simulink model "sim"  (R2020a)
settings: Solver=VariableStepAuto  StartTime=0.0  StopTime=10.0  RelTol=1e-3
undefined symbols (not defined in the file): A, An, B, Bn, C, K_lqr, Ln, P_0, Q_n, R_n, Ts, x_0, x_kalman
libraries: simulink_extras x2
settings Model: Creator=Artis  LastModifiedBy=Artis

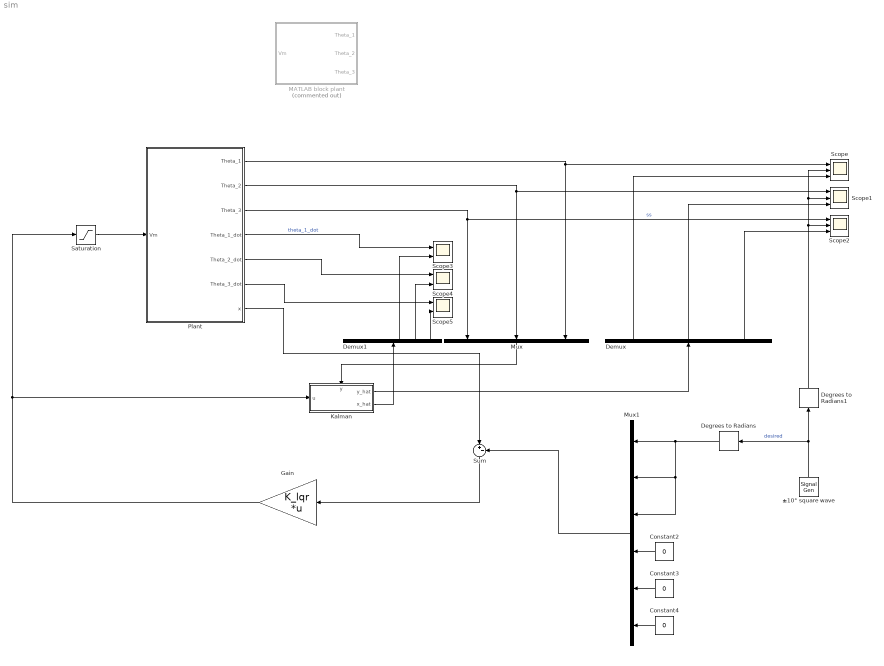
== system sim ==
  Constant2 : Constant  Value=0
  Constant3 : Constant  Value=0
  Constant4 : Constant  Value=0
  Degrees to Radians : simulink_extras/Transformations/Degrees to Radians
  Degrees to Radians1 : simulink_extras/Transformations/Degrees to Radians
  Demux : Demux  Outputs=3
  Demux1 : Demux  Outputs=6
  Gain : Gain  Gain=K_lqr  Multiplication=Matrix(K*u) (u vector)
  Kalman : Subsystem
      settings: PortSchema="{\"entries\":[{\"content\":{\"sides\":[{\"content\":{\"connectorIds\":[\"In1\"]},\"type\":\"ConnectorPlacement.EquallySpacedRectSide\",\"uuid\":\"62bff884-1764-4624-86bb-c0f466d25cc0\"},{\"content\":{\"connectorIds\":[\"Out1\",\"Out2\"],\"side\":\"RIGHT\"},\"type\":\"ConnectorPlacement.EquallySpacedRectSide\",\"uuid\":\"eceabb9a-6e11-42f6-82ff-ae26c39c3440\"},{\"content\":{\"connectorIds\":[\"In2\"],\"side\":\"TOP\"},\"type\":\"ConnectorPlacement.EquallySpacedRectSide\",\"uuid\":\"6bdeda42-7cc5-45d4-ac99-29c27164ef4c\"}]},\"type\":\"ConnectorPlacement.EquallySpacedConnector\",\"uuid\":\"cdaf1b78-b767-40c4-a6aa-db1d943e4267\"}],\"packageUris\":[\"http://schema.mathworks.com/mf0/Connector/19700101\"],\"version\":\"1.0\"}"
  MATLAB block plant : Subsystem  Commented=on
  Mux : Mux  Inputs=3
  Mux1 : Mux  Inputs=6
  Plant : Subsystem
  Saturation : Saturate  UpperLimit=6  LowerLimit=-6
  Scope : Scope  NumInputPorts=3
  Scope1 : Scope  NumInputPorts=3
  Scope2 : Scope  NumInputPorts=3
  Scope3 : Scope  NumInputPorts=2
  Scope4 : Scope  NumInputPorts=2
  Scope5 : Scope  NumInputPorts=2
  Sum : Sum  Inputs=|+-
  ±10° square wave : SignalGenerator  WaveForm=square  Amplitude=10  Units=rad/sec
  wires:
  Plant/1(Theta_1) -> Scope/1, Mux/3
  Plant/2(Theta_2) -> Mux/2, Scope1/1
  Plant/3(Theta_3) -> Mux/1, Scope2/1  "ss"
  Gain/1 -> Kalman/1(u), Saturation/1
  ±10° square wave/1 -> Degrees to Radians1/1, Degrees to Radians/1  "desired"
  Mux/1 -> Kalman/2(y)
  Kalman/1(y_hat) -> Demux/1
  Demux/1 -> Scope/3
  Demux/2 -> Scope1/3
  Demux/3 -> Scope2/3
  Plant/4(Theta_1_dot) -> Scope3/1  "theta_1_dot"
  Plant/5(Theta_2_dot) -> Scope4/1
  Plant/6(Theta_3_dot) -> Scope5/1
  Demux1/4 -> Scope3/2
  Demux1/5 -> Scope4/2
  Demux1/6 -> Scope5/2
  Kalman/2(x_hat) -> Demux1/1
  Sum/1 -> Gain/1
  Mux1/1 -> Sum/2
  Constant2/1 -> Mux1/4
  Constant3/1 -> Mux1/5
  Constant4/1 -> Mux1/6
  Plant/7(x) -> Sum/1
  Degrees to Radians/1 -> Mux1/3, Mux1/2, Mux1/1
  Saturation/1 -> Plant/1(Vm)
  Degrees to Radians1/1 -> Scope/2, Scope1/2, Scope2/2

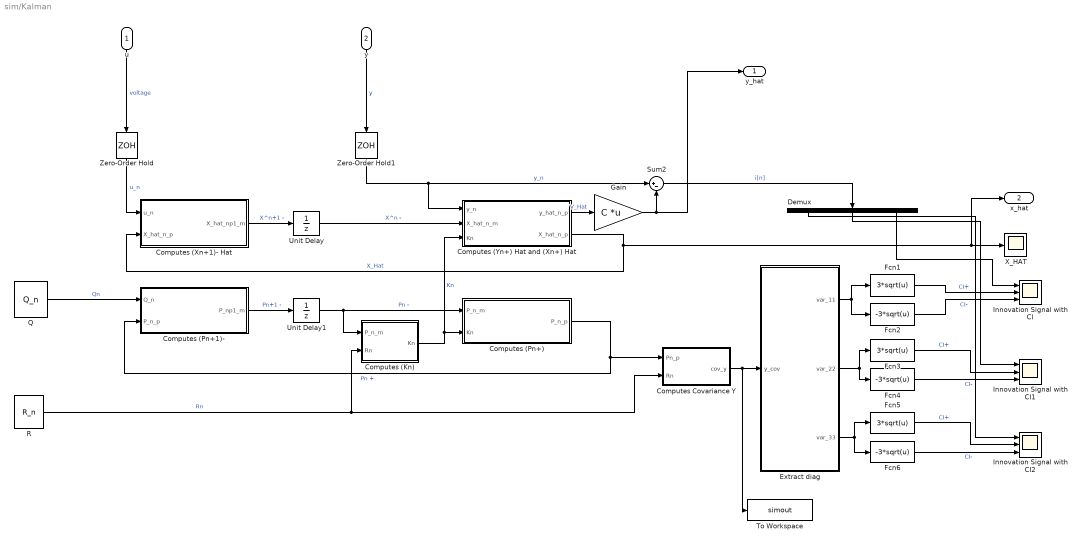
== system sim/Kalman ==
  u : Inport
  y : Inport  Port=2
  Computes (Kn) : MATLAB Function  TreatAsAtomicUnit=on
  Computes (Pn+) : MATLAB Function  TreatAsAtomicUnit=on
  "Computes (Pn+1)- " : MATLAB Function  TreatAsAtomicUnit=on
  Computes (Xn+1)- Hat : MATLAB Function  TreatAsAtomicUnit=on
  Computes (Yn+) Hat and (Xn+) Hat : MATLAB Function  TreatAsAtomicUnit=on
  Computes Covariance Y : MATLAB Function  TreatAsAtomicUnit=on
  Demux : Demux  Outputs=3
  Extract diag : MATLAB Function  TreatAsAtomicUnit=on
  Fcn1 : Fcn  Expr=3*sqrt(u)
  Fcn2 : Fcn  Expr=-3*sqrt(u)
  Fcn3 : Fcn  Expr=3*sqrt(u)
  Fcn4 : Fcn  Expr=-3*sqrt(u)
  Fcn5 : Fcn  Expr=3*sqrt(u)
  Fcn6 : Fcn  Expr=-3*sqrt(u)
  Gain : Gain  Gain=C  Multiplication=Matrix(K*u) (u vector)
  Innovation Signal with CI : Scope  NumInputPorts=3
  Innovation Signal with CI1 : Scope  NumInputPorts=3
  Innovation Signal with CI2 : Scope  NumInputPorts=3
  Q : Constant  Value=Q_n
  R : Constant  Value=R_n
  Sum2 : Sum  Inputs=|+-
  To Workspace : ToWorkspace  VariableName=simout  SampleTime=-1
  Unit Delay : UnitDelay  InitialCondition=x_kalman  SampleTime=Ts  HasFrameUpgradeWarning=on
  Unit Delay1 : UnitDelay  InitialCondition=P_0  SampleTime=Ts  HasFrameUpgradeWarning=on
  X_HAT : Scope
  Zero-Order Hold : ZeroOrderHold  SampleTime=Ts
  Zero-Order Hold1 : ZeroOrderHold  SampleTime=Ts
  y_hat : Outport
  x_hat : Outport  Port=2
  wires:
  Zero-Order Hold/1 -> Computes (Xn+1)- Hat/1(u_n)  "u_n"
  Fcn2/1 -> Innovation Signal with CI/3  "CI-"
  Unit Delay1/1 -> Computes (Pn+)/1(P_n_m), Computes (Kn)/1(P_n_m)  "Pn -"
  Computes (Xn+1)- Hat/1(X_hat_np1_m) -> Unit Delay/1  "X^n+1 -"
  R/1 -> Computes (Kn)/2(Rn), Computes Covariance Y/2(Rn)  "Rn"
  Computes (Kn)/1(Kn) -> Computes (Yn+) Hat and (Xn+) Hat/3(Kn), Computes (Pn+)/2(Kn)  "Kn"
  Fcn1/1 -> Innovation Signal with CI/2  "CI+"
  Sum2/1 -> Demux/1  "i[n]"
  u/1 -> Zero-Order Hold/1  "voltage"
  Computes (Yn+) Hat and (Xn+) Hat/1(y_hat_n_p) -> Gain/1  "V_Hat"
  Unit Delay/1 -> Computes (Yn+) Hat and (Xn+) Hat/2(X_hat_n_m)  "X^n -"
  Zero-Order Hold1/1 -> Computes (Yn+) Hat and (Xn+) Hat/1(y_n), Sum2/1  "y_n"
  "Computes (Pn+1)- "/1(P_np1_m) -> Unit Delay1/1  "Pn+1 -"
  Computes (Yn+) Hat and (Xn+) Hat/2(X_hat_n_p) -> Computes (Xn+1)- Hat/2(X_hat_n_p), x_hat/1, X_HAT/1  "X_Hat"
  Q/1 -> "Computes (Pn+1)- "/1(Q_n)  "Qn"
  Computes (Pn+)/1(P_n_p) -> Computes Covariance Y/1(Pn_p), "Computes (Pn+1)- "/2(P_n_p)  "Pn +"
  y/1 -> Zero-Order Hold1/1  "y"
  Computes Covariance Y/1(cov_y) -> To Workspace/1, Extract diag/1(y_cov)
  Gain/1 -> y_hat/1, Sum2/2
  Demux/3 -> Innovation Signal with CI/1
  Extract diag/1(var_11) -> Fcn2/1, Fcn1/1
  Extract diag/2(var_22) -> Fcn3/1, Fcn4/1
  Fcn3/1 -> Innovation Signal with CI1/2  "CI+"
  Fcn4/1 -> Innovation Signal with CI1/3  "CI-"
  Demux/2 -> Innovation Signal with CI1/1
  Fcn6/1 -> Innovation Signal with CI2/3  "CI-"
  Fcn5/1 -> Innovation Signal with CI2/2  "CI+"
  Extract diag/3(var_33) -> Fcn6/1, Fcn5/1
  Demux/1 -> Innovation Signal with CI2/1

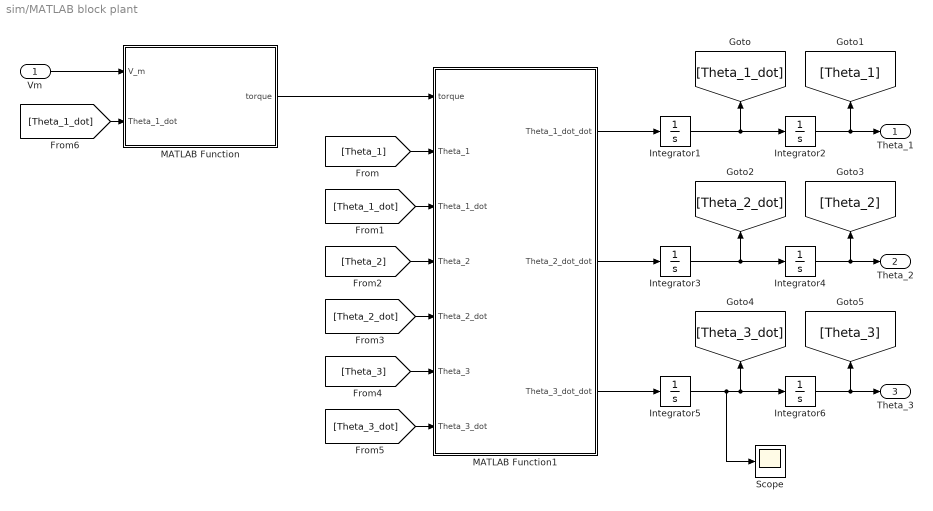
== system sim/MATLAB block plant ==
  Vm : Inport
  Integrator{1..6} (6 alike) : Integrator
  MATLAB Function : MATLAB Function  TreatAsAtomicUnit=on
  MATLAB Function1 : MATLAB Function  TreatAsAtomicUnit=on
  Scope : Scope
  Theta_1 : Outport
  Theta_2 : Outport  Port=2
  Theta_3 : Outport  Port=3
  wires:
  Vm/1 -> MATLAB Function/1(V_m)
  MATLAB Function/1(torque) -> MATLAB Function1/1(torque)
  Integrator1/1 -> Integrator2/1, [Theta_1_dot]
  MATLAB Function1/1(Theta_1_dot_dot) -> Integrator1/1
  Integrator2/1 -> [Theta_1], Theta_1/1
  [Theta_1] -> MATLAB Function1/2(Theta_1)
  [Theta_1_dot] -> MATLAB Function1/3(Theta_1_dot)
  [Theta_2_dot] -> MATLAB Function1/5(Theta_2_dot)
  [Theta_2] -> MATLAB Function1/4(Theta_2)
  [Theta_3] -> MATLAB Function1/6(Theta_3)
  [Theta_3_dot] -> MATLAB Function1/7(Theta_3_dot)
  Integrator4/1 -> [Theta_2], Theta_2/1
  Integrator3/1 -> Integrator4/1, [Theta_2_dot]
  MATLAB Function1/2(Theta_2_dot_dot) -> Integrator3/1
  MATLAB Function1/3(Theta_3_dot_dot) -> Integrator5/1
  Integrator5/1 -> Scope/1, Integrator6/1, [Theta_3_dot]
  Integrator6/1 -> [Theta_3], Theta_3/1
  [Theta_1_dot] -> MATLAB Function/2(Theta_1_dot)

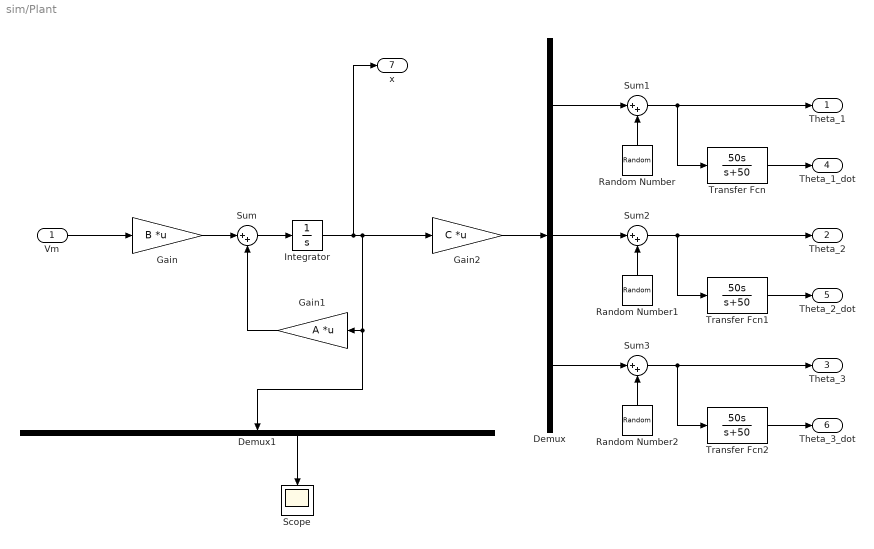
== system sim/Plant ==
  Vm : Inport
  Demux : Demux  Outputs=3
  Demux1 : Demux  Outputs=6
  Gain : Gain  Gain=B  Multiplication=Matrix(K*u) (u vector)
  Gain1 : Gain  Gain=A  Multiplication=Matrix(K*u) (u vector)
  Gain2 : Gain  Gain=C  Multiplication=Matrix(K*u) (u vector)
  Integrator : Integrator  InitialCondition=x_0
  Random Number : RandomNumber  Variance=1e-3  SampleTime=Ts
  Random Number1 : RandomNumber  Variance=1e-3  Seed=1  SampleTime=Ts
  Random Number2 : RandomNumber  Variance=1e-3  Seed=2  SampleTime=Ts
  Scope : Scope
  Sum{,1..3} (4 alike) : Sum  Inputs=|++
  Transfer Fcn : TransferFcn  Numerator=[50 0]  Denominator=[1 50]
  Transfer Fcn1 : TransferFcn  Numerator=[50 0]  Denominator=[1 50]
  Transfer Fcn2 : TransferFcn  Numerator=[50 0]  Denominator=[1 50]
  Theta_1 : Outport
  Theta_2 : Outport  Port=2
  Theta_3 : Outport  Port=3
  Theta_1_dot : Outport  Port=4
  Theta_2_dot : Outport  Port=5
  Theta_3_dot : Outport  Port=6
  x : Outport  Port=7
  wires:
  Gain/1 -> Sum/1
  Sum/1 -> Integrator/1
  Integrator/1 -> Gain2/1, Demux1/1, Gain1/1, x/1
  Gain1/1 -> Sum/2
  Gain2/1 -> Demux/1
  Demux/1 -> Sum1/1
  Vm/1 -> Gain/1
  Sum1/1 -> Transfer Fcn/1, Theta_1/1
  Transfer Fcn/1 -> Theta_1_dot/1
  Random Number/1 -> Sum1/2
  Transfer Fcn1/1 -> Theta_2_dot/1
  Random Number1/1 -> Sum2/2
  Sum2/1 -> Theta_2/1, Transfer Fcn1/1
  Demux/2 -> Sum2/1
  Sum3/1 -> Theta_3/1, Transfer Fcn2/1
  Random Number2/1 -> Sum3/2
  Transfer Fcn2/1 -> Theta_3_dot/1
  Demux/3 -> Sum3/1
  Demux1/4 -> Scope/1

== matlab function sim/MATLAB block plant/MATLAB Function1 ==
  data: torque input; Theta_1_dot_dot output; Theta_2_dot_dot output; Theta_1 input; Theta_1_dot input; Theta_2 input; Theta_2_dot input; Theta_3 input; Theta_3_dot input; Theta_3_dot_dot output
function [Theta_1_dot_dot, Theta_2_dot_dot, Theta_3_dot_dot]= fcn(torque, Theta_1, Theta_1_dot, Theta_2, Theta_2_dot, Theta_3, Theta_3_dot)
B_1 = 0.015;
B_2 = 0.0015;
J_1 = 0.0022;
J_2 = 0.000545;
B_3 = B_2;
J_3 = J_2;

K_s1 = 1;
K_s2 = K_s1;

Theta_1_dot_dot = (torque-B_1*Theta_1_dot-K_s1*(Theta_1-Theta_2))/J_1;
Theta_2_dot_dot = (-B_2*Theta_2_dot-K_s1*(Theta_2-Theta_1)-K_s2*(Theta_2-Theta_3))/J_2;
Theta_3_dot_dot = (-B_3*Theta_3_dot-K_s2*(Theta_3-Theta_2))/J_3;

== matlab function sim/MATLAB block plant/MATLAB Function ==
  data: V_m input; torque output; Theta_1_dot input
function torque = fcn(V_m, Theta_1_dot)
k_t = 0.00767;
k_m = 0.00767;
R_m = 2.6;
nu_m = 0.69;
nu_g = 0.85;
K_gi = 14;
K_ge_low = 1;
K_ge_high = 5;
K_g = (K_gi*K_ge_low*K_ge_high);
torque = (nu_g*K_g*k_t*(V_m-K_g*k_m*Theta_1_dot))/R_m;

== matlab function sim/Kalman/Computes (Pn+1)-  ==
  data: Q_n input; P_n_p input; P_np1_m output; An parameter; Ln parameter
function P_np1_m = fcn(Q_n,P_n_p,An, Ln)

P_np1_m = An*P_n_p*An' + Ln*Q_n*Ln';

== matlab function sim/Kalman/Computes (Pn+) ==
  data: P_n_m input; P_n_p output; Kn input; Hn parameter
function P_n_p = fcn(P_n_m,Kn,Hn)
P_n_p=P_n_m-Kn*Hn*P_n_m;

== matlab function sim/Kalman/Computes (Kn) ==
  data: P_n_m input; Kn output; Rn input; Hn parameter
function Kn = fcn(P_n_m,Rn,Hn)

Kn=P_n_m*Hn'/(Hn*P_n_m*Hn'+Rn);

== matlab function sim/Kalman/Computes (Xn+1)- Hat ==
  data: u_n input; X_hat_n_p input; X_hat_np1_m output; An parameter; Bn parameter
function X_hat_np1_m = fcn(u_n,X_hat_n_p, An, Bn)

X_hat_np1_m= An*X_hat_n_p + Bn*u_n;

== matlab function sim/Kalman/Computes (Yn+) Hat and (Xn+) Hat ==
  data: y_hat_n_p output; y_n input; X_hat_n_m input; X_hat_n_p output; Kn input; Hn parameter
function [y_hat_n_p,X_hat_n_p] = fcn(y_n,X_hat_n_m,Kn,Hn)
X_hat_n_p=X_hat_n_m+Kn*(y_n-Hn*X_hat_n_m);

y_hat_n_p=X_hat_n_p;

== matlab function sim/Kalman/Computes Covariance Y ==
  data: Pn_p input; cov_y output; Rn input; Hn parameter
function cov_y = fcn(Pn_p,Rn, Hn)

cov_y= Hn * Pn_p * Hn'+ Rn;

== matlab function sim/Kalman/Extract diag ==
  data: y_cov input; var_11 output; var_22 output; var_33 output
function [var_11, var_22, var_33]= fcn(y_cov)
var_11 = y_cov(1,1);
var_22 = y_cov(2,2);
var_33 = y_cov(3,3);
